simulink model "blun"  (Simulink 8.5)
settings: Solver=ode45  SolverMode=SingleTasking  StartTime=0.0  StopTime=6  MaxStep=.002  RelTol=1e-3  AbsTol=1e-6
settings Model: Creator=PC  LastModifiedBy=PC  ExtModeTrigMode=oneshot  ExtModeArmWhenConnect=off
settings DataIOCC: LimitDataPoints=off
settings OptimizationCC: BlockReduction=off  BooleanDataType=off  ExpressionDepthLimit=128
settings DebuggingCC: SaveWithParameterizedLinksMsg=none  SignalResolutionControl=TryResolveAllWithWarning  MultiTaskDSMMsg=warning  MultiTaskCondExecSysMsg=none  FcnCallInpInsideContextMsg=EnableAllAsError  StateNameClashWarn=none
settings HardwareCC: TargetUnknown=on

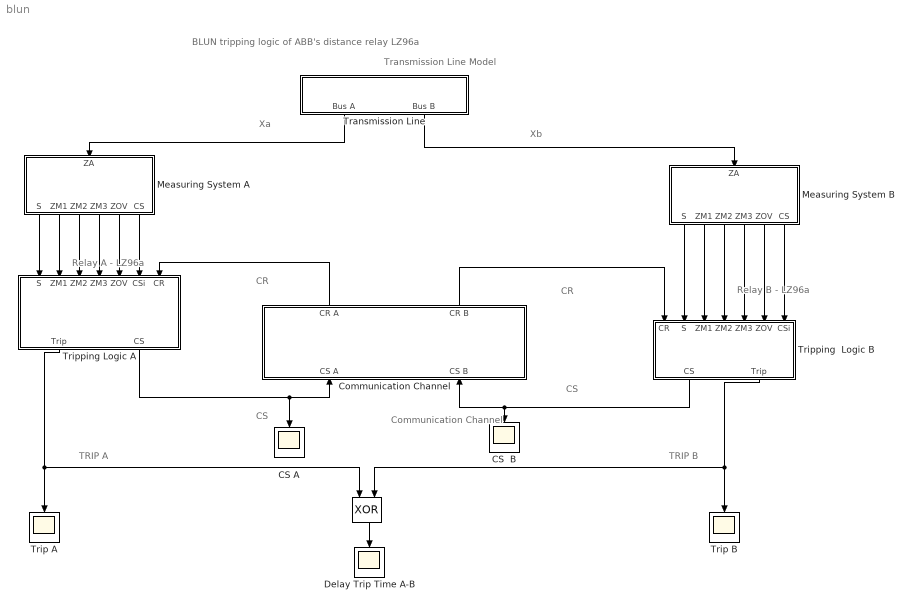
== system blun ==
  note: Transmission Line Model
  note: Relay A - LZ96a
  note: Xa
  note: Xb
  note: CS
  note: CS
  note: CR
  note: CR
  note: TRIP A
  note: TRIP B
  note: BLUN tripping logic of ABB's distance relay LZ96a
  note: Relay B - LZ96a
  note: Communication
      | Channel
  " " : Logic  Operator=XOR
  " Tripping Logic A" : Subsystem
  " Tripping  Logic B" : Subsystem
  CS  B : Scope
      settings: TickLabels=on  YMin=-0.5  YMax=2
  CS A : Scope
      settings: TickLabels=on  YMin=-0.5  YMax=2
  Communication Channel : Subsystem  mask(Communication channel.){Tdelay=0, failure=off, err_signal=0}
      mask prompts: Tdelay "Channel delay time [ms]:"; failure "Communication channel failure."; err_signal "Erroneous signal:"
      mask TypeOptions err_signal: 0 | 1
  Delay Trip Time A-B : Scope
      settings: TickLabels=on  YMin=-0.5  YMax=2
  Measuring System A : Subsystem  mask(Measuring system - starter block){ZM=[0.8 1.7 2.6], Tzone=[0 .5 0.8], ZOV=1.7, S=[-1 3], Tstarter=1.0, ZMB=-1.9, tHF=0.2}
      mask prompts: ZM "Zone reach [z1 z2  z3]  [p.u.]:"; Tzone "Zone times [z1 z2  z3]  [s]:"; ZOV "Overreach zone [pu]"; S "Starter range [Smin Smax] [p.u.]:"; Tstarter "Starter time [s]:"; ZMB "ZMB [pu.]:"; tHF "THF [s]"
  Measuring System B : Subsystem  mask(Measuring system - starter block){ZM=[0.8 1.7 2.6], Tzone=[0 .5 0.8], ZOV=1.7, S=[-1 3], Tstarter=1.0, ZMB=-1.9, tHF=0.2}
      mask prompts: ZM "Zone reach [z1 z2  z3]  [p.u.]:"; Tzone "Zone times [z1 z2  z3]  [s]:"; ZOV "Overreach Zone [pu]"; S "Starter range [Smin Smax] [p.u.]:"; Tstarter "Starter time [s]:"; ZMB "ZMB [pu.]:"; tHF "thf [s]:"
  Transmission Line : Subsystem  mask(Model of transmission line with fault){x=0.5, Tfault=0.1}
      mask prompts: x "Fault location from bus A [p.u.]"; Tfault "Fault time [s]:"
  Trip A : Scope
      settings: TickLabels=on  YMin=-0.5  YMax=2
  Trip B : Scope
      settings: TickLabels=on  YMin=-0.5  YMax=2
  wires:
  Transmission Line/2(Bus B) -> Measuring System B/1(ZA)
  " "/1 -> Delay Trip Time A-B/1
  Measuring System A/6(CS) -> " Tripping Logic A"/6(CSi)
  Transmission Line/1(Bus A) -> Measuring System A/1(ZA)
  " Tripping Logic A"/1(Trip) -> Trip A/1, " "/1
  Measuring System B/1("S ") -> " Tripping  Logic B"/2(S)
  Measuring System B/3("ZM2 ") -> " Tripping  Logic B"/4(ZM2)
  Measuring System B/4("ZM3 ") -> " Tripping  Logic B"/5(ZM3)
  Measuring System B/5("ZOV ") -> " Tripping  Logic B"/6("ZOV ")
  Measuring System B/6(CS) -> " Tripping  Logic B"/7(CSi)
  Measuring System B/2("ZM1 ") -> " Tripping  Logic B"/3(ZM1)
  " Tripping  Logic B"/2(Trip) -> Trip B/1, " "/2
  Communication Channel/1(CR A) -> " Tripping Logic A"/7(CR)
  " Tripping  Logic B"/1(CS) -> Communication Channel/2(CS B), CS  B/1
  " Tripping Logic A"/2(CS) -> Communication Channel/1(CS A), CS A/1
  Communication Channel/2(CR B) -> " Tripping  Logic B"/1(CR)
  Measuring System A/5("ZOV ") -> " Tripping Logic A"/5("ZOV ")
  Measuring System A/4("ZM3 ") -> " Tripping Logic A"/4(ZM3)
  Measuring System A/3("ZM2 ") -> " Tripping Logic A"/3(ZM2)
  Measuring System A/2("ZM1 ") -> " Tripping Logic A"/2(ZM1)
  Measuring System A/1("S ") -> " Tripping Logic A"/1(S)

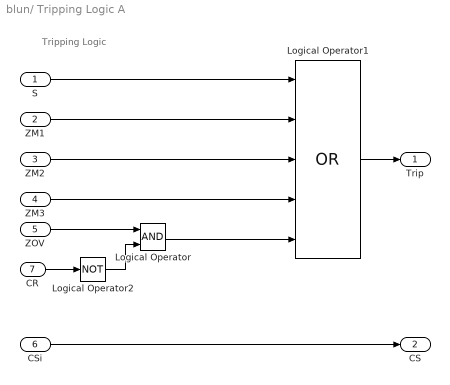
== system blun/ Tripping Logic A ==
  note: Tripping Logic
  S : Inport
  ZM1 : Inport  Port=2
  ZM2 : Inport  Port=3
  ZM3 : Inport  Port=4
  "ZOV " : Inport  Port=5
  CSi : Inport  Port=6
  CR : Inport  Port=7
  Logical Operator : Logic
  Logical Operator1 : Logic  Operator=OR  Inputs=5
  Logical Operator2 : Logic  Operator=NOT  Inputs=1
  Trip : Outport  InitialOutput=0
  CS : Outport  Port=2  InitialOutput=0
  wires:
  CSi/1 -> CS/1
  "ZOV "/1 -> Logical Operator/1
  Logical Operator2/1 -> Logical Operator/2
  CR/1 -> Logical Operator2/1
  Logical Operator/1 -> Logical Operator1/5
  ZM3/1 -> Logical Operator1/4
  ZM2/1 -> Logical Operator1/3
  ZM1/1 -> Logical Operator1/2
  S/1 -> Logical Operator1/1
  Logical Operator1/1 -> Trip/1

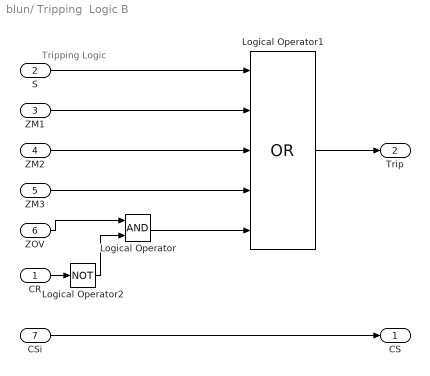
== system blun/ Tripping  Logic B ==
  note: Tripping Logic
  CR : Inport
  S : Inport  Port=2
  ZM1 : Inport  Port=3
  ZM2 : Inport  Port=4
  ZM3 : Inport  Port=5
  "ZOV " : Inport  Port=6
  CSi : Inport  Port=7
  Logical Operator : Logic
  Logical Operator1 : Logic  Operator=OR  Inputs=5
  Logical Operator2 : Logic  Operator=NOT  Inputs=1
  CS : Outport  InitialOutput=0
  Trip : Outport  Port=2  InitialOutput=0
  wires:
  Logical Operator2/1 -> Logical Operator/2
  Logical Operator1/1 -> Trip/1
  CR/1 -> Logical Operator2/1
  CSi/1 -> CS/1
  "ZOV "/1 -> Logical Operator/1
  S/1 -> Logical Operator1/1
  ZM1/1 -> Logical Operator1/2
  ZM2/1 -> Logical Operator1/3
  ZM3/1 -> Logical Operator1/4
  Logical Operator/1 -> Logical Operator1/5

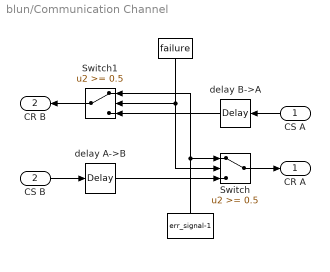
== system blun/Communication Channel ==
  CS A : Inport
  CS B : Inport  Port=2
  " " : Constant  Value=failure
  "  " : Constant  Value=err_signal-1
  Switch : Switch  Threshold=0.5  SaturateOnIntegerOverflow=on  InputSameDT=on
  Switch1 : Switch  Threshold=0.5  SaturateOnIntegerOverflow=on  InputSameDT=on
  delay A->B : TransportDelay  DelayTime=Tdelay/1000+1e-12
  delay B->A : TransportDelay  DelayTime=Tdelay/1000+1e-12
  CR A : Outport  InitialOutput=0
  CR B : Outport  Port=2  InitialOutput=0
  wires:
  Switch/1 -> CR A/1
  CS B/1 -> delay A->B/1
  CS A/1 -> delay B->A/1
  Switch1/1 -> CR B/1
  "  "/1 -> Switch1/1, Switch/1
  delay A->B/1 -> Switch/3
  delay B->A/1 -> Switch1/3
  " "/1 -> Switch/2, Switch1/2

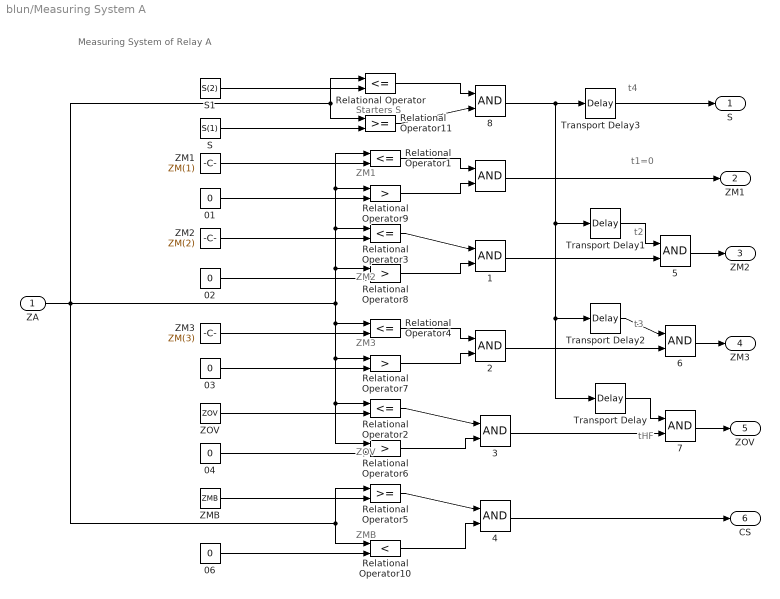
== system blun/Measuring System A ==
  note: Measuring System of Relay A
  note: Starters S
  note: ZM2
  note: ZOV
  note: ZM1
  note: ZM3
  note: ZMB
  note: t4
  note: t1=0
  note: t2
  note: t3
  note: tHF
  ZA : Inport
   {,1..8} (9 alike) : Logic
  01 : Constant  Value=0
  02 : Constant  Value=0
  03 : Constant  Value=0
  04 : Constant  Value=0
  06 : Constant  Value=0
  Relational Operator{,1..4} (5 alike) : RelationalOperator  Operator=<=  InputSameDT=on
  Relational Operator10 : RelationalOperator  Operator=<  InputSameDT=on
  Relational Operator11 : RelationalOperator  InputSameDT=on
  Relational Operator5 : RelationalOperator  InputSameDT=on
  Relational Operator{6..9} (4 alike) : RelationalOperator  Operator=>  InputSameDT=on
  S : Constant  Value=S(1)
  S1 : Constant  Value=S(2)
  Transport Delay : TransportDelay  DelayTime=tHF
  Transport Delay1 : TransportDelay  DelayTime=Tzone(2)
  Transport Delay2 : TransportDelay  DelayTime=Tzone(3)
  Transport Delay3 : TransportDelay  DelayTime=Tstarter
  ZM1 : Constant  Value=ZM(1)
  ZM2 : Constant  Value=ZM(2)
  ZM3 : Constant  Value=ZM(3)
  ZMB : Constant  Value=ZMB
  ZOV : Constant  Value=ZOV
  "S " : Outport  InitialOutput=0
  "ZM1 " : Outport  Port=2  InitialOutput=0
  "ZM2 " : Outport  Port=3  InitialOutput=0
  "ZM3 " : Outport  Port=4  InitialOutput=0
  "ZOV " : Outport  Port=5  InitialOutput=0
  CS : Outport  Port=6  InitialOutput=0
  wires:
  ZM2/1 -> Relational Operator3/2
  ZA/1 -> Relational Operator1/1, Relational Operator9/1, Relational Operator3/1, Relational Operator8/1, Relational Operator6/1, Relational Operator2/1, Relational Operator7/1, Relational Operator4/1, Relational Operator5/1, Relational Operator10/1, Relational Operator/1, Relational Operator11/1
  Relational Operator3/1 -> " 1"/1
  Relational Operator8/1 -> " 1"/2
  Relational Operator9/1 -> " "/2
  Relational Operator1/1 -> " "/1
  01/1 -> Relational Operator9/2
  ZM1/1 -> Relational Operator1/2
  ZM3/1 -> Relational Operator4/2
  ZOV/1 -> Relational Operator2/2
  Relational Operator2/1 -> " 3"/1
  Relational Operator6/1 -> " 3"/2
  04/1 -> Relational Operator6/2
  Relational Operator4/1 -> " 2"/1
  03/1 -> Relational Operator7/2
  Relational Operator7/1 -> " 2"/2
  06/1 -> Relational Operator10/2
  ZMB/1 -> Relational Operator5/2
  Relational Operator5/1 -> " 4"/1
  Relational Operator10/1 -> " 4"/2
  " 4"/1 -> CS/1
  02/1 -> Relational Operator8/2
  Transport Delay3/1 -> "S "/1
  " "/1 -> "ZM1 "/1
  Transport Delay1/1 -> " 5"/1
  " 5"/1 -> "ZM2 "/1
  " 1"/1 -> " 5"/2
  Transport Delay2/1 -> " 6"/1
  " 6"/1 -> "ZM3 "/1
  " 2"/1 -> " 6"/2
  Transport Delay/1 -> " 7"/1
  " 3"/1 -> " 7"/2
  S1/1 -> Relational Operator/2
  S/1 -> Relational Operator11/2
  " 7"/1 -> "ZOV "/1
  " 8"/1 -> Transport Delay3/1, Transport Delay1/1, Transport Delay2/1, Transport Delay/1
  Relational Operator11/1 -> " 8"/2
  Relational Operator/1 -> " 8"/1

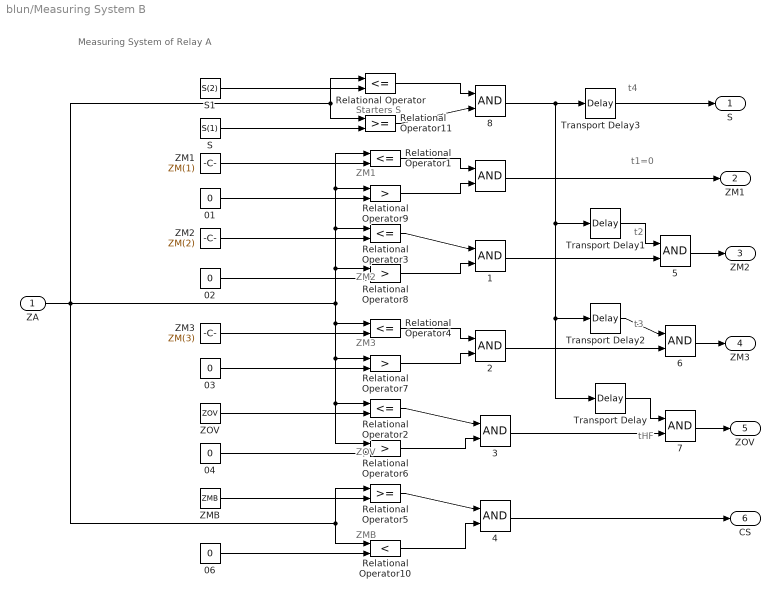
== system blun/Measuring System B ==
  note: Measuring System of Relay A
  note: Starters S
  note: ZM2
  note: ZOV
  note: ZM1
  note: ZM3
  note: ZMB
  note: t4
  note: t1=0
  note: t2
  note: t3
  note: tHF
  ZA : Inport
   {,1..8} (9 alike) : Logic
  01 : Constant  Value=0
  02 : Constant  Value=0
  03 : Constant  Value=0
  04 : Constant  Value=0
  06 : Constant  Value=0
  Relational Operator{,1..4} (5 alike) : RelationalOperator  Operator=<=  InputSameDT=on
  Relational Operator10 : RelationalOperator  Operator=<  InputSameDT=on
  Relational Operator11 : RelationalOperator  InputSameDT=on
  Relational Operator5 : RelationalOperator  InputSameDT=on
  Relational Operator{6..9} (4 alike) : RelationalOperator  Operator=>  InputSameDT=on
  S : Constant  Value=S(1)
  S1 : Constant  Value=S(2)
  Transport Delay : TransportDelay  DelayTime=tHF
  Transport Delay1 : TransportDelay  DelayTime=Tzone(2)
  Transport Delay2 : TransportDelay  DelayTime=Tzone(3)
  Transport Delay3 : TransportDelay  DelayTime=Tstarter
  ZM1 : Constant  Value=ZM(1)
  ZM2 : Constant  Value=ZM(2)
  ZM3 : Constant  Value=ZM(3)
  ZMB : Constant  Value=ZMB
  ZOV : Constant  Value=ZOV
  "S " : Outport  InitialOutput=0
  "ZM1 " : Outport  Port=2  InitialOutput=0
  "ZM2 " : Outport  Port=3  InitialOutput=0
  "ZM3 " : Outport  Port=4  InitialOutput=0
  "ZOV " : Outport  Port=5  InitialOutput=0
  CS : Outport  Port=6  InitialOutput=0
  wires:
  ZM2/1 -> Relational Operator3/2
  ZA/1 -> Relational Operator1/1, Relational Operator9/1, Relational Operator3/1, Relational Operator8/1, Relational Operator6/1, Relational Operator2/1, Relational Operator7/1, Relational Operator4/1, Relational Operator5/1, Relational Operator10/1, Relational Operator/1, Relational Operator11/1
  Relational Operator3/1 -> " 1"/1
  Relational Operator8/1 -> " 1"/2
  Relational Operator9/1 -> " "/2
  Relational Operator1/1 -> " "/1
  01/1 -> Relational Operator9/2
  ZM1/1 -> Relational Operator1/2
  ZM3/1 -> Relational Operator4/2
  ZOV/1 -> Relational Operator2/2
  Relational Operator2/1 -> " 3"/1
  Relational Operator6/1 -> " 3"/2
  04/1 -> Relational Operator6/2
  Relational Operator4/1 -> " 2"/1
  03/1 -> Relational Operator7/2
  Relational Operator7/1 -> " 2"/2
  06/1 -> Relational Operator10/2
  ZMB/1 -> Relational Operator5/2
  Relational Operator5/1 -> " 4"/1
  Relational Operator10/1 -> " 4"/2
  " 4"/1 -> CS/1
  02/1 -> Relational Operator8/2
  Transport Delay3/1 -> "S "/1
  " "/1 -> "ZM1 "/1
  Transport Delay1/1 -> " 5"/1
  " 5"/1 -> "ZM2 "/1
  " 1"/1 -> " 5"/2
  Transport Delay2/1 -> " 6"/1
  " 6"/1 -> "ZM3 "/1
  " 2"/1 -> " 6"/2
  Transport Delay/1 -> " 7"/1
  " 3"/1 -> " 7"/2
  S1/1 -> Relational Operator/2
  S/1 -> Relational Operator11/2
  " 7"/1 -> "ZOV "/1
  " 8"/1 -> Transport Delay3/1, Transport Delay1/1, Transport Delay2/1, Transport Delay/1
  Relational Operator11/1 -> " 8"/2
  Relational Operator/1 -> " 8"/1

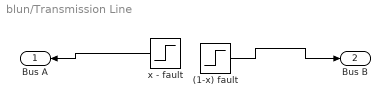
== system blun/Transmission Line ==
  (1-x) fault : Step  Time=Tfault  Before=1000  After=1-x  SampleTime=0
  x - fault : Step  Time=Tfault  Before=1000  After=x  SampleTime=0
  Bus A : Outport  InitialOutput=0
  Bus B : Outport  Port=2  InitialOutput=0
  wires:
  (1-x) fault/1 -> Bus B/1
  x - fault/1 -> Bus A/1
